simulink model "HT_ctrl_MFAC"  (R2023a)
settings: Solver=VariableStepAuto  StartTime=0.0  StopTime=40  FixedStep=1  RelTol=1e-3
undefined symbols (not defined in the file): D1, Delta
libraries: spsThreePhaseParallelRLCLoadLib x3, spsExcitationSystemModel x2, spsThreePhaseSourceLib x1, spsSynchronousMachinepuStandardLib x1, spsThreePhaseBreakerLib x1, spsThreePhaseTransformerTwoWindingsLib x1, spsVoltageMeasurementLib x1, spsGroundLib x1, sps_lib x1
settings Model: Creator=zzzaa  LastModifiedBy=HP
settings OptimizationCC: ReuseModelBlockBuffer=off

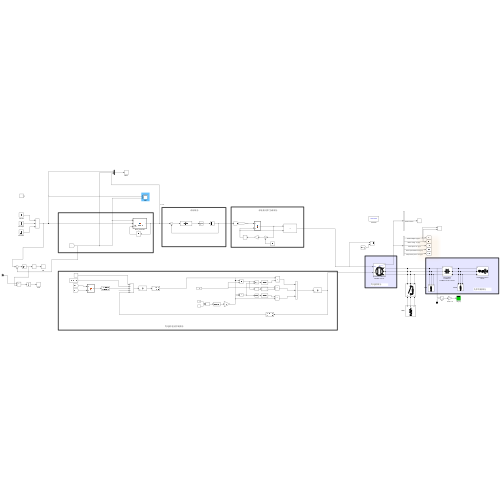
[thumbnail: Simulink's stored preview of the top-level diagram]
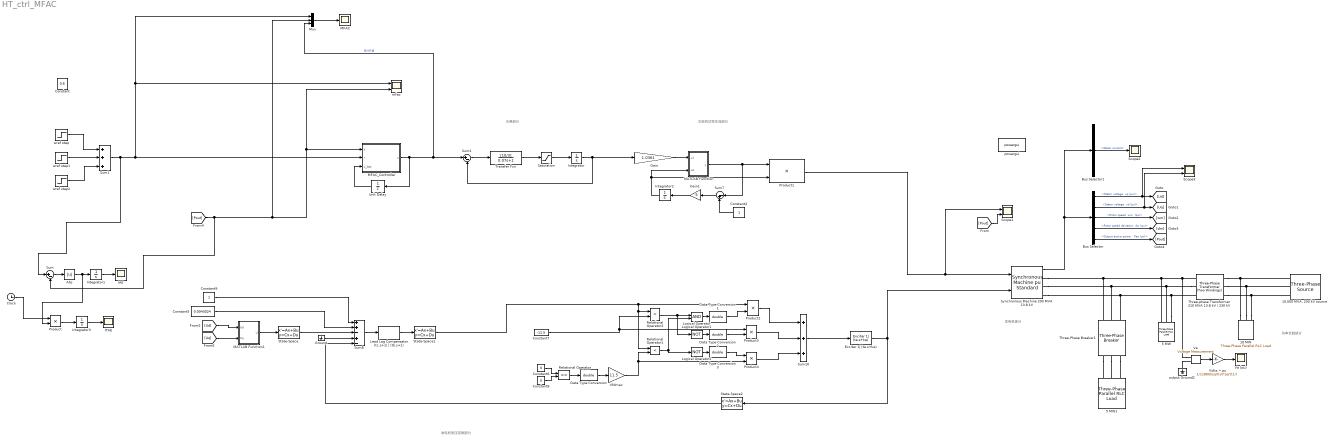
== system HT_ctrl_MFAC ==
  note: 水轮机功率生成部分
  note: 水闸部分
  note: 发电机电压控制部分
  note: 发电机部分
  note: 功率负载部分
  10 MW : spsThreePhaseParallelRLCLoadLib/Three-Phase Parallel RLC Load  LConnTagsString=A|B|C  Configuration=Y (grounded)  NominalVoltage=230e3  Vabc=[1e3 1e3 1e3]  Vabcp=[1e3 1e3 1e3]  NominalFrequency=60  UnbalancedPower=off  ActivePower=10000000  InductivePower=0  CapacitivePower=0  Pabc=[10e3 9e3 11e3]  QLabc=[100 90 110]  QCabc=[100 90 110]  Pabcp=[10e3 9e3 11e3]  QLabcp=[100 90 110]  QCabcp=[100 90 110]  Measurements=None  LoadType=constant Z
  "10,000 MVA, 230 kV source" : spsThreePhaseSourceLib/Three-Phase Source  InternalConnection=Yg  VoltagePhases=off  Voltage=(230000)*1.00006  PhaseAngle=-0.77547  Voltage_phases=[25e3 25e3 25e3]/sqrt(3)  PhaseAngles_phases=[0 -120 +120]  Frequency=60  NonIdealSource=on  SpecifyImpedance=on  Resistance=0.529  Inductance=0.0140  ShortCircuitLevel=10000e6  BaseVoltage=230e3  XRratio=10  BusType=swing  Pref=0  Qref=0  Prefabc=[10e3, 10e3, 10e3]  Qrefabc=[0, 0, 0]  Qmin=-Inf  Qmax=Inf
  5 MW : spsThreePhaseParallelRLCLoadLib/Three-Phase Parallel RLC Load  LConnTagsString=A|B|C  Configuration=Y (grounded)  NominalVoltage=13.8e3  Vabc=[1e3 1e3 1e3]  Vabcp=[1e3 1e3 1e3]  NominalFrequency=60  UnbalancedPower=off  ActivePower=5000000  InductivePower=0  CapacitivePower=0  Pabc=[10e3 9e3 11e3]  QLabc=[100 90 110]  QCabc=[100 90 110]  Pabcp=[10e3 9e3 11e3]  QLabcp=[100 90 110]  QCabcp=[100 90 110]  Measurements=None  LoadType=constant Z
  5 MW1 : spsThreePhaseParallelRLCLoadLib/Three-Phase Parallel RLC Load  LConnTagsString=A|B|C  Configuration=Y (grounded)  NominalVoltage=13.8e3  Vabc=[1e3 1e3 1e3]  Vabcp=[1e3 1e3 1e3]  NominalFrequency=60  UnbalancedPower=off  ActivePower=3000000  InductivePower=0  CapacitivePower=0  Pabc=[10e3 9e3 11e3]  QLabc=[100 90 110]  QCabc=[100 90 110]  Pabcp=[10e3 9e3 11e3]  QLabcp=[100 90 110]  QCabcp=[100 90 110]  Measurements=None  LoadType=constant Z
  Abs : Abs  SaturateOnIntegerOverflow=off
  Bus Selector : BusSelector  OutputSignals="dq0 components.Stator voltage  vq (pu),dq0 components.Stator voltage  vd (pu),Mechanical.Rotor speed  wm  (pu),Mechanical.Rotor speed deviation  dw (pu),Output active power   Peo (pu)"
  Bus Selector1 : BusSelector  OutputSignals=Stator current
  Clock : Clock
  Constant : Constant  Value=0.6
  Constant4 : Constant
  Constant5 : Constant  Value=0.0043024
  Constant6 : Constant  Value=0
  Constant7 : Constant  Value=-11.5
  Constant8 : Constant  Value=0
  Constant9 : Constant
  Data Type Conversion{,1..3} (4 alike) : DataTypeConversion  OutDataTypeStr=double  SaturateOnIntegerOverflow=off  RndMeth=Floor
  Exciter 1| (te.s+ke) : spsExcitationSystemModel/Continuous/Exciter 1| (te.s+ke)  N=1  D=[0 1]  Y0=1.2907  U0=1.2907
  Gain : Gain  Gain=1.0361
  Gain1 : Gain  Gain=5
  Ground : Ground
  IAE : Scope
  ITAE : Scope
  Integrator : Integrator  InitialCondition=0.72544  LimitOutput=on  UpperSaturationLimit=0.97518  LowerSaturationLimit=0.01
  Integrator1 : Integrator
  Integrator2 : Integrator  InitialCondition=0.75161
  Integrator3 : Integrator
  Lead Lag Compensator (tc.s+1) | (tb.s+1) : spsExcitationSystemModel/Continuous/Lead Lag Compensator (tc.s+1) | (tb.s+1)  N=[0 1]  D=[0 1]  Y0=0.0043024  U0=0.0043024
  Logical Operator : Logic
  Logical Operator1 : Logic  Operator=NOT  Inputs=1
  Logical Operator2 : Logic  Operator=NOT  Inputs=1
  MATLAB Function : MATLAB Function  TreatAsAtomicUnit=on
  MATLAB Function1 : MATLAB Function  TreatAsAtomicUnit=on
  MFAC : Scope
  MFAC_Controller : MATLAB Function  TreatAsAtomicUnit=on  SystemSampleTime=0.01
  Mux : Mux  Inputs=3
  Product : Product
  Product1 : Product
  Product2 : Product  InputSameDT=on  SaturateOnIntegerOverflow=on  OutDataTypeStr=Inherit: Same as first input
  Product3 : Product  InputSameDT=on  SaturateOnIntegerOverflow=on  OutDataTypeStr=Inherit: Same as first input
  Product4 : Product  InputSameDT=on  SaturateOnIntegerOverflow=on  OutDataTypeStr=Inherit: Same as first input
  Relational Operator : RelationalOperator  Operator===
  Relational Operator1 : RelationalOperator  Operator=<
  Relational Operator2 : RelationalOperator  Operator=>
  Saturation : Saturate  UpperLimit=0.1  LowerLimit=-0.1
  Scope1 : Scope  NumInputPorts=2
  Scope2 : Scope
  Scope3 : Scope  NumInputPorts=2
  State-Space : StateSpace  A=-50  C=50  D=0  InitialCondition=0.02
  State-Space1 : StateSpace  A=-1000  C=300000  D=0  InitialCondition=4.3024e-6
  State-Space2 : StateSpace  A=-10  C=-0.1  D=0.01  InitialCondition=0.1297
  Sum : Sum  Inputs=|+-
  Sum1 : Sum  Inputs=+++  InputSameDT=on  SaturateOnIntegerOverflow=on  OutDataTypeStr=Inherit: Same as first input
  Sum10 : Sum  Inputs=+++  InputSameDT=on  SaturateOnIntegerOverflow=on  OutDataTypeStr=Inherit: Same as first input
  Sum2 : Sum  Inputs=|+-
  Sum7 : Sum  Inputs=|-+
  Sum8 : Sum  Inputs=++-+-  InputSameDT=on  SaturateOnIntegerOverflow=on  OutDataTypeStr=Inherit: Same as first input
  Synchronous Machine 200 MVA 13.8 kV : spsSynchronousMachinepuStandardLib/Synchronous Machine pu Standard  PresetModel=No  MechanicalLoad=Mechanical power Pm  ShowDetailedParameters=on  RotorType=Salient-pole  Units=per unit standard parameters  MeasurementBus=off  NominalParameters="[ 200E6  13800   60 ]"  Reactances1=[ 31 32 33 34 35 36 37 ]  Reactances2=[ 1.305, 0.296, 0.252, 0.474, 0.243, 0.18 ]  dAxisTimeConstants=Short-circuit  qAxisTimeConstants=Open-circuit  TimeConstants1=[]  TimeConstants2=[]  TimeConstants3=[]  TimeConstants4=[]  TimeConstants5=[ 1.01, 0.053, 0.1 ]  TimeConstants6=[]  TimeConstants7=[]  TimeConstants8=[]  StatorResistance=2.8544e-3  Mechanical=[ 3.2 0 2]  PolePairs=2  InitialConditions=[0 -94.2826 0.750185 0.750185 0.750185 -24.943 -144.943 95.057 1.29071]  SetSaturation=off  Saturation=[0.6404,0.7127,0.8441,0.9214,0.9956,1.082,1.19,1.316,1.457;0.7,0.7698,0.8872,0.9466,0.9969,1.046,1.1,1.151,1.201]  LoadFlowParameters=[1 150000000 0 0]  TsPowergui=0  TsBlock=-1  IterativeModel=Trapezoidal non iterative  IterativeDiscreteModel=Trapezoidal non iterative  BusType=PV  Pref=150000000  Qref=0  Qmin=-Inf  Qmax=Inf  PLF=0  QLF=0
  Three-Phase Breaker1 : spsThreePhaseBreakerLib/Three-Phase Breaker  InitialState=open  SwitchA=on  SwitchB=on  SwitchC=on  SwitchTimes=[30]  External=off  BreakerResistance=0.01  SnubberResistance=1e6  SnubberCapacitance=inf  Measurements=None
  Three-phase Transformer 210 MVA 13.8 kV / 230 kV : spsThreePhaseTransformerTwoWindingsLib/Three-Phase Transformer (Two Windings)  Winding1Connection=Delta (D1)  Winding2Connection=Yg  CoreType=Three single-phase transformers  SetSaturation=off  Hysteresis=off  DataFile='hysteresis'  SetInitialFlux=off  Measurements=None  UNITS=pu  NominalPower=[ 210e6 60 ]  Winding1="[ 13.8e3 0.0027  0.08]"  Winding2=[ 230e3 0.0027 0.08]  Rm=500  Lm=500  L0=0.5  Saturation="[ 0,0  ;  0.005,1.2  ;  1.0,1.4 ]"  InitialFluxes=[ 0.8 , -0.8 , 0.7 ]  BreakLoop=off  DiscreteSolver=Trapezoidal iterative  DataType=off  TransfoNumber=0
  Transfer Fcn : TransferFcn  Numerator=[10/3]  Denominator=[0.07 1]
  Unit Delay : UnitDelay  SampleTime=0.01  HasFrameUpgradeWarning=on
  Va : spsVoltageMeasurementLib/Voltage Measurement  Tag=PoWeRsYsTeMmEaSuReMeNt  PhasorSimulation=off  OutputType=Magnitude  PSBequivalent=0
  Va (pu) : Scope
  Vfdmax : Gain  Gain=11.5  SaturateOnIntegerOverflow=on  OutDataTypeStr=Inherit: Same as input  ParamDataTypeStr=Inherit: Same as input
  Volts > pu : Gain  Gain=1/(13800/sqrt(3)*sqrt(2))  SaturateOnIntegerOverflow=on  OutDataTypeStr=Inherit: Same as input  ParamDataTypeStr=Inherit: Same as input
  mfac : Scope  NumInputPorts=2
  output Ground2 : spsGroundLib/Ground  LConnTagsString=a
  powergui : sps_lib/powergui  Priority=2  SimulationMode=Continuous  SampleTime=0  frequency=60  Iterations=50  frequencyindice=60  Pbase=100e6  ErrMax=0.0001  UnitsV=kV  UnitsW=MW  buscounter=0  FunctionMessages=off  echomessages=off  EnableUseOfTLC=off  CurrentSourceSwitches=off  DisableSnubberDevices=off  DisableRonSwitches=off  DisableVfSwitches=off  DisplayEquations=off  AutomaticDiscreteSolvers=off  SolverType=Tustin  Interpol=off  ExternalGateDelay=off  methode=off  Ts=0  x0status=blocks  SPID=on  SwTol=0  HookPort=off  NonlinearTolerance=0  nMaxIteration=15  ContinueOnMaxIteration=off  RestoreLinks=warning  ResistiveCurrentMeasurement=off  Frange=logspace(0,3,50)  Ylog=off  Xlog=off  ShowGrid=off  save=off  variable=ZData  structure=0  ZoomFFT=on  StartTime=0.0  cycles=2  DisplayStyle=off  fundamental=60  FreqAxis=off  MaxFrequency=1000  frequencyindicesteady=1  RmsSteady=1  display=off
  wref step : Step  Time=0  After=0.5  SampleTime=0
  wref step1 : Step  Time=20  After=0.25  SampleTime=0
  wref step2 : Step  Time=35  After=0.15  SampleTime=0
  wires:
  Va/1 -> Volts > pu/1
  Volts > pu/1 -> Va (pu)/1
  Synchronous Machine 200 MVA 13.8 kV/1 -> Bus Selector1/1, Bus Selector/1
  Bus Selector/1 -> Scope3/1, [Ud]  "<Stator voltage  vq (pu)>"
  Bus Selector/2 -> Scope3/2, [Uq]  "<Stator voltage  vd (pu)>"
  Bus Selector/3 -> [wm]  "<Rotor speed  wm  (pu)>"
  Bus Selector/4 -> [dm]  "<Rotor speed deviation  dw (pu)>"
  Bus Selector/5 -> [Pout]  "<Output active power   Peo (pu)>"
  [Pout] -> Mux/2, mfac/2, MFAC_Controller/1(y), Sum/2
  MFAC_Controller/1(u) -> Unit Delay/1, Mux/3, Sum2/1  "导叶开度"
  Transfer Fcn/1 -> Saturation/1
  Saturation/1 -> Integrator/1
  Sum2/1 -> Transfer Fcn/1
  Gain/1 -> MATLAB Function/1(u1)
  MATLAB Function/1(y) -> Product1/1, Sum7/1
  Constant4/1 -> Sum7/2
  Sum7/1 -> Gain1/1
  Gain1/1 -> Integrator2/1
  Integrator2/1 -> MATLAB Function/2(u2), Product1/2
  State-Space2/1 -> Sum8/5
  Exciter 1| (te.s+ke)/1 -> Synchronous Machine 200 MVA 13.8 kV/2, State-Space2/1
  MATLAB Function1/1(U) -> State-Space/1
  Lead Lag Compensator (tc.s+1) | (tb.s+1)/1 -> State-Space1/1
  [Ud] -> MATLAB Function1/1(Ud)
  Constant5/1 -> Sum8/2
  Constant9/1 -> Sum8/1
  Sum10/1 -> Exciter 1| (te.s+ke)/1
  [Uq] -> MATLAB Function1/2(Uq)
  Sum8/1 -> Lead Lag Compensator (tc.s+1) | (tb.s+1)/1
  Ground/1 -> Sum8/4
  Logical Operator2/1 -> Data Type Conversion3/1
  State-Space/1 -> Sum8/3
  Constant6/1 -> Relational Operator/1
  Product2/1 -> Sum10/1
  Constant8/1 -> Relational Operator/2
  Product4/1 -> Sum10/3
  Relational Operator1/1 -> Logical Operator2/1, Logical Operator/2
  Product3/1 -> Sum10/2
  Constant7/1 -> Product3/1, Relational Operator2/2
  Relational Operator2/1 -> Logical Operator1/1, Logical Operator/1
  Logical Operator/1 -> Data Type Conversion1/1
  Vfdmax/1 -> Product4/2, Relational Operator1/2
  State-Space1/1 -> Product2/1, Relational Operator1/1, Relational Operator2/1
  Data Type Conversion/1 -> Vfdmax/1
  Data Type Conversion1/1 -> Product2/2
  Data Type Conversion2/1 -> Product3/2
  Logical Operator1/1 -> Data Type Conversion2/1
  Data Type Conversion3/1 -> Product4/1
  Relational Operator/1 -> Data Type Conversion/1
  Product1/1 -> Scope1/1, Synchronous Machine 200 MVA 13.8 kV/1
  Bus Selector1/1 -> Scope2/1  "<Stator current>"
  [Pout] -> Scope1/2
  wref step/1 -> Sum1/1
  wref step1/1 -> Sum1/2
  wref step2/1 -> Sum1/3
  Mux/1 -> MFAC/1
  Sum1/1 -> Sum/1, mfac/1, Mux/1, MFAC_Controller/2(r)
  Integrator/1 -> Sum2/2, Gain/1
  Sum/1 -> Abs/1
  Abs/1 -> Product/2, Integrator1/1
  Integrator1/1 -> IAE/1
  Clock/1 -> Product/1
  Product/1 -> Integrator3/1
  Integrator3/1 -> ITAE/1
  Unit Delay/1 -> MFAC_Controller/3(u_last)
  connections:
  10 MW/LConn2 -- Three-phase Transformer 210 MVA 13.8 kV / 230 kV/RConn2 -- "10,000 MVA, 230 kV source"/RConn2
  Va/LConn1 -- Three-Phase Breaker1/LConn1 -- Synchronous Machine 200 MVA 13.8 kV/RConn1 -- 5 MW/LConn1 -- Three-phase Transformer 210 MVA 13.8 kV / 230 kV/LConn1
  10 MW/LConn3 -- Three-phase Transformer 210 MVA 13.8 kV / 230 kV/RConn3 -- "10,000 MVA, 230 kV source"/RConn3
  10 MW/LConn1 -- Three-phase Transformer 210 MVA 13.8 kV / 230 kV/RConn1 -- "10,000 MVA, 230 kV source"/RConn1
  5 MW/LConn3 -- Three-Phase Breaker1/LConn3 -- Synchronous Machine 200 MVA 13.8 kV/RConn3 -- Three-phase Transformer 210 MVA 13.8 kV / 230 kV/LConn3
  Three-phase Transformer 210 MVA 13.8 kV / 230 kV/LConn2 -- Synchronous Machine 200 MVA 13.8 kV/RConn2 -- Three-Phase Breaker1/LConn2 -- 5 MW/LConn2
  output Ground2/LConn1 -- Va/LConn2
  Three-Phase Breaker1/RConn3 -- 5 MW1/LConn3
  Three-Phase Breaker1/RConn2 -- 5 MW1/LConn2
  Three-Phase Breaker1/RConn1 -- 5 MW1/LConn1

== matlab function HT_ctrl_MFAC/MATLAB Function1 ==
  data: Ud input; U output; Uq input
function U = fcn(Ud, Uq)

U = sqrt(Ud^2+Uq^2);

== matlab function HT_ctrl_MFAC/MATLAB Function ==
  data: u1 input; y output; u2 input
function y = fcn(u1,u2)

y = (u2/u1)^2;

end

== matlab function HT_ctrl_MFAC/MFAC_Controller ==
  data: y input; r input; u output; u_last input
function u = mfac_ctrl(y, r, u_last)
%#codegen
% 4端口:
% 输入:  y, r, u_last
% 输出:  u
%
% 特点:
% 1) 不依赖精确模型
% 2) 只在线估计伪偏导phi，稳定性比全参数在线辨识更好
% 3) 参考软化 + 增量限幅 + 幅值限幅 + 死区抑振
% 4) 适合作为毕业设计里的“自编预测/自适应控制器”

persistent y1 y2
persistent u1 u2
persistent phi
persistent r_f
persistent inited

if isempty(inited)
    y1 = 0;
    y2 = 0;
    u1 = 0;
    u2 = 0;

    % 伪偏导初值：表示“u增加，y大概率也增加”
    % 如果你的对象是反向作用，后面把它改成负数
    phi = 0.15;

    % 平滑参考初值
    r_f = 0;

    inited = true;
end

%% ===== 参数区（先给你一版保守的） =====
% 参考软化
alpha_r = 0.10;      % 越小越平缓，先保守一点

% 主控制增益
rho = 0.35;          % 主步长，太大容易振荡

% 自适应正则
lambda = 1.20;       % 越大越稳，越小越快

% 伪偏导更新参数
eta = 0.08;          % phi更新步长
mu  = 0.10;          % 防止分母过小

% 约束
u_min  = -1.15;
u_max  =  1.15;
du_min = -0.035;
du_max =  0.035;

% 死区，小误差时减少抖动
e_dead = 0.003;

% phi限制，防止数值跑飞
phi_min_abs = 0.02;
phi_max_abs = 2.0;

% 控制平滑因子
beta_u = 0.25;       % 0~1，越大越保守

%% ===== 1) 参考软化 =====
r_f = (1 - alpha_r) * r_f + alpha_r * r;

%% ===== 2) 误差 =====
e = r_f - y;

if abs(e) < e_dead
    e = 0;
end

%% ===== 3) 在线更新伪偏导 phi =====
dy = y - y1;
du_prev = u1 - u2;

den_phi = mu + du_prev * du_prev;
phi = phi + eta * du_prev * (dy - phi * du_prev) / den_phi;

% 防止phi漂移到0附近或发散
if abs(phi) < phi_min_abs
    if phi >= 0
        phi = phi_min_abs;
    else
        phi = -phi_min_abs;
    end
end

if abs(phi) > phi_max_abs
    if phi >= 0
        phi = phi_max_abs;
    else
        phi = -phi_max_abs;
    end
end

%% ===== 4) 自适应控制增益 =====
% 误差大 -> 稍积极；误差小 -> 稍平缓
rho_eff = rho * (1 + 0.8 * min(abs(e), 0.5));

%% ===== 5) 增量控制律 =====
% 一步预测思想:
% y(k+1) ≈ y(k) + phi * Δu(k)
% 令未来输出向参考靠近，得到增量控制律
du_raw = rho_eff * phi * e / (lambda + phi * phi);

% 控制平滑
du = beta_u * du_raw;

%% ===== 6) 增量限幅 =====
if du > du_max
    du = du_max;
elseif du < du_min
    du = du_min;
end

%% ===== 7) 输出限幅 =====
u = u_last + du;

if u > u_max
    u = u_max;
elseif u < u_min
    u = u_min;
end

%% ===== 8) 更新历史量 =====
y2 = y1;
y1 = y;

u2 = u1;
u1 = u_last;
